simulink library "lib_Convection_FCSphere"  (R2015a)
settings: Solver=ode45  StartTime=0.0  StopTime=10.0  RelTol=1e-3
libraries: simulink x2
settings Model: Creator=jlkratz  LastModifiedBy=jlkratz

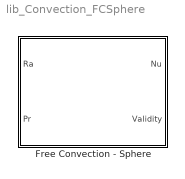
== system lib_Convection_FCSphere ==
  Free Convection - Sphere : Subsystem  mask(TSAT: Sphere Free Convection){}
      mask help: This block estimates the average Nusselt number of a free convecting flow about a sphere. The employed correlation was recommended by Churchill. The Rayliegh number should be calculated using the diameter of the sphere as the characteristic length. Note that all fluid properrties should be evaluated at film temperature (average of the bulk fluid and surface temperatures).
      mask Help: web(which('Convection_TSAT_FCSphere.html'),'-helpbrowser')

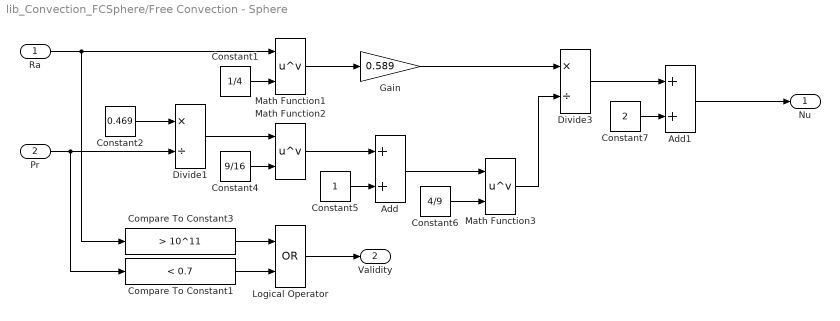
== system lib_Convection_FCSphere/Free Convection - Sphere ==
  Ra : Inport
  Pr : Inport  Port=2
  Add : Sum
  Add1 : Sum
  Compare To Constant1 : simulink/Logic and Bit Operations/Compare To Constant  relop=<  const=0.7  OutDataTypeStr=boolean
  Compare To Constant3 : simulink/Logic and Bit Operations/Compare To Constant  relop=>  const=10^11  OutDataTypeStr=boolean
  Constant1 : Constant  Value=1/4
  Constant2 : Constant  Value=0.469
  Constant4 : Constant  Value=9/16
  Constant5 : Constant
  Constant6 : Constant  Value=4/9
  Constant7 : Constant  Value=2
  Divide1 : Product  Inputs=*/
  Divide3 : Product  Inputs=*/
  Gain : Gain  Gain=0.589
  Logical Operator : Logic  Operator=OR  AllPortsSameDT=off  OutDataTypeStr=boolean
  Math Function1 : Math  Operator=pow  SaturateOnIntegerOverflow=on
  Math Function2 : Math  Operator=pow  SaturateOnIntegerOverflow=on
  Math Function3 : Math  Operator=pow  SaturateOnIntegerOverflow=on
  Nu : Outport
  Validity : Outport  Port=2
  wires:
  Compare To Constant1/1 -> Logical Operator/2
  Logical Operator/1 -> Validity/1
  Compare To Constant3/1 -> Logical Operator/1
  Add1/1 -> Nu/1
  Constant7/1 -> Add1/2
  Divide3/1 -> Add1/1
  Math Function3/1 -> Divide3/2
  Gain/1 -> Divide3/1
  Constant6/1 -> Math Function3/2
  Add/1 -> Math Function3/1
  Constant5/1 -> Add/2
  Math Function2/1 -> Add/1
  Constant4/1 -> Math Function2/2
  Divide1/1 -> Math Function2/1
  Constant2/1 -> Divide1/1
  Math Function1/1 -> Gain/1
  Constant1/1 -> Math Function1/2
  Pr/1 -> Divide1/2, Compare To Constant1/1
  Ra/1 -> Math Function1/1, Compare To Constant3/1
